simulink model "rtwdemo_sfexprfold"  (Simulink 7.6)
settings: Solver=ode5  StartTime=0.0  StopTime=10.0  RelTol=1e-3  SampleTimeConstraint=STIndependent
PreLoadFcn:
  | rtwdemo_sfexprfold_data
undefined symbols (not defined in the file or in its folder): LOWER, T1Break, T1Data, T2Data, UPPER
libraries: rtwdemowidgets x2
Description:
  | Expression Folding Between Simulink(R) and Stateflow(R)
settings Model: Creator=The MathWorks Inc.  ExtModeAutoUpdateStatusClock=off
settings DataIOCC: SaveOutput=off  SaveTime=off  SignalLoggingName=sigsOut
settings OptimizationCC: InlineParams=on  InlineInvariantSignals=on  StateBitsets=on  DataBitsets=on  UseTempVars=on  EfficientFloat2IntCast=on  EfficientMapNaN2IntZero=off
settings DebuggingCC: CheckExecutionContextPreStartOutputMsg=on  CheckExecutionContextRuntimeOutputMsg=on  SolverPrmCheckMsg=none  StrictBusMsg=ErrorOnBusTreatedAsVector
settings HardwareCC: ProdIntDivRoundTo=Zero  ProdEndianess=LittleEndian  ProdHWDeviceType=Generic->32-bit Embedded Processor  TargetHWDeviceType=Generic->32-bit Embedded Processor
settings SFSimCC: SimParseCustomCode=off
settings RTWCC: TLCOptions=-p0 -aWarnNonSaturatedBlocks=0  GenerateReport=on  RTWVerbose=off  ProcessScript=grt_make_rtw_hook  LaunchReport=on
settings CodeAppCC: ForceParamTrailComments=on
settings GRTTargetCC: TargetFcnLib=ansi_tfl_tmw.mat

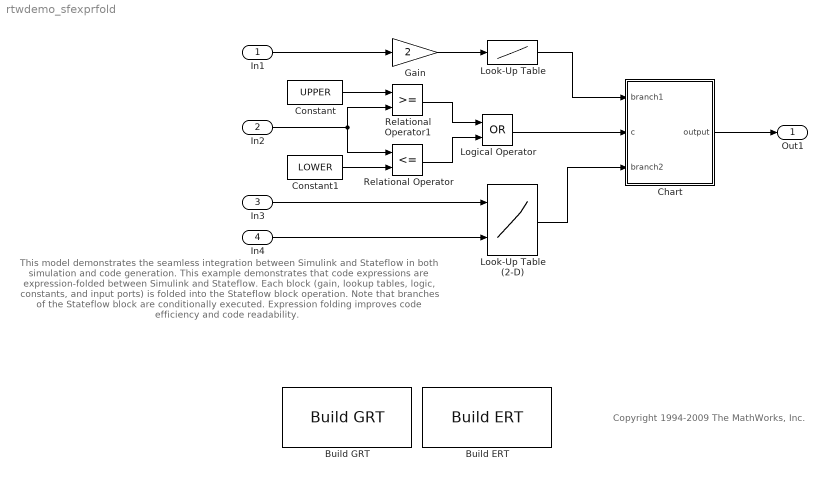
== system rtwdemo_sfexprfold ==
  note: This model demonstrates the seamless integration between Simulink and Stateflow in both
      | simulation and code generation.  This example demonstrates that code expressions are
      | expression-folded between Simulink and Stateflow.  Each block (gain, lookup tables,
      | logic, constants, and input ports) is folded into the Stateflow block operation. Note that
      | branches of the Stateflow block are conditionally executed. Expression folding improves
      | code efficiency and code readability.
  note: Copyright 1994-2009 The MathWorks, Inc.
  In1 : Inport  OutDataTypeStr=double  PortDimensions=1
  In2 : Inport  Port=2  OutDataTypeStr=double  PortDimensions=1
  In3 : Inport  Port=3  OutDataTypeStr=double  PortDimensions=1
  In4 : Inport  Port=4  OutDataTypeStr=double  PortDimensions=1
  Build ERT : rtwdemowidgets/Build ERT  SystemSampleTime=-1  attrib_overrides={}
  Build GRT : rtwdemowidgets/Build GRT  SystemSampleTime=-1  attrib_overrides={}
  Chart : Stateflow chart  TreatAsAtomicUnit=on
  Constant : Constant  Value=UPPER
  Constant1 : Constant  Value=LOWER
  Gain : Gain  Gain=2  SaturateOnIntegerOverflow=on  OutDataTypeStr=Inherit: Same as input  ParamDataTypeStr=Inherit: Same as input
  Logical Operator : Logic  Operator=OR
  Look-Up Table : Lookup  InputValues=T1Break  Table=T1Data  SaturateOnIntegerOverflow=on
  Look-Up Table (2-D) : Lookup2D  RowIndex=T2Break  ColumnIndex=T2Break  Table=T2Data  InputSameDT=on
  Relational Operator : RelationalOperator  Operator=<=  InputSameDT=on
  Relational Operator1 : RelationalOperator  InputSameDT=on
  Out1 : Outport
  wires:
  Relational Operator1/1 -> Logical Operator/1
  Relational Operator/1 -> Logical Operator/2
  Logical Operator/1 -> Chart/2(c)
  Constant1/1 -> Relational Operator/2
  In1/1 -> Gain/1
  Gain/1 -> Look-Up Table/1
  Look-Up Table (2-D)/1 -> Chart/3(branch2)
  Constant/1 -> Relational Operator1/1
  In2/1 -> Relational Operator1/2, Relational Operator/1
  In3/1 -> Look-Up Table (2-D)/1
  In4/1 -> Look-Up Table (2-D)/2
  Look-Up Table/1 -> Chart/1(branch1)
  Chart/1(output) -> Out1/1

== stateflow chart Chart ==
  note: This chart is acting as an if-else condition.
      | Using a Simulink switch or if-action block
      | results in virtually identical code.
  (junction 5) -> (junction 4) [order 1] : [c]{output = branch1;}
  (default) -> (junction 5)
  (junction 5) -> (junction 4) [order 2] : {output = branch2;}
  data: branch1 input double size=1; c input boolean size=1; branch2 input double size=1; output output double size=1
